simulink model "signals"  (R2023a)
settings: Solver=VariableStepAuto  StartTime=0.0  StopTime=inf  RelTol=1e-3
settings Model: Creator=siril  LastModifiedBy=siril

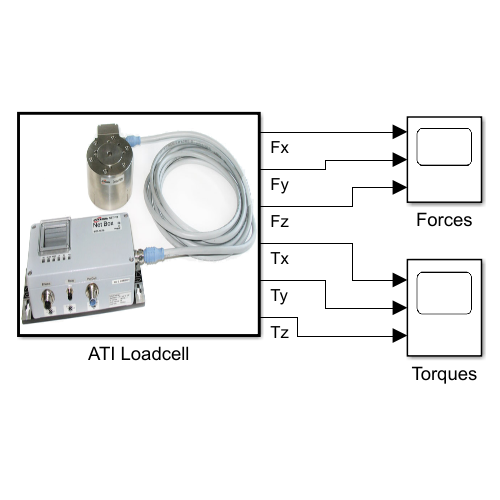
[thumbnail: Simulink's stored preview of the top-level diagram]
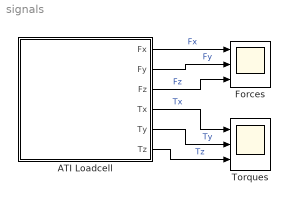
== system signals ==
  ATI Loadcell : MATLAB Function  TreatAsAtomicUnit=on
  Forces : Scope  NumInputPorts=3
  Torques : Scope  NumInputPorts=3
  wires:
  ATI Loadcell/1(Fx) -> Forces/1  "Fx"
  ATI Loadcell/2(Fy) -> Forces/2  "Fy"
  ATI Loadcell/3(Fz) -> Forces/3  "Fz"
  ATI Loadcell/4(Tx) -> Torques/1  "Tx"
  ATI Loadcell/5(Ty) -> Torques/2  "Ty"
  ATI Loadcell/6(Tz) -> Torques/3  "Tz"

== matlab function signals/ATI Loadcell ==
  data: Fx output; Fy output; Fz output; Tx output; Ty output; Tz output
function [Fx, Fy, Fz, Tx, Ty, Tz] = netFT_readData()
    % Declare the extrinsic wrapper function
    coder.extrinsic('myWrapper');  % Tell Simulink that myWrapper is an external function

    % Initialize output variables as numeric types
    Fx = 0;
    Fy = 0;
    Fz = 0;
    Tx = 0;
    Ty = 0;
    Tz = 0;

    % Call the wrapper function
    [Fx, Fy, Fz, Tx, Ty, Tz] = myWrapper();  % Get the force and torque data
end
